simulink model "Q1Induction_Motor"  (R2013a)
settings: Solver=ode45  StartTime=0.0  StopTime=5  MaxStep=1e-4  RelTol=1e-3
settings Model: Creator=Sony  LastModifiedBy=Sony

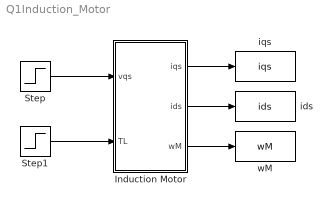
== system Q1Induction_Motor ==
  Induction Motor : Subsystem  mask{Rs=0.277, Lr=0.05606, Ls=0.0553, Lm=0.0538, La=0.0553-((0.0538*0.0538)/0.05606), J=0.0165, B=0.05, ws=2*pi*60, P=4}
      mask prompts: Rs "Rs (ohm)"; Lr "Lr (H)"; Ls "Ls (H)"; Lm "Lm (H)"; La "La (H)"; J "J (kgm^2)"; B "B (kgm^2/s)"; ws "ws (rad/s)"
  Step : Step  Time=0.1  After=200*sqrt(2)/sqrt(3)  SampleTime=0
  Step1 : Step  Time=2.5  SampleTime=0
  ids : ToWorkspace  VariableName=ids  SampleTime=-1  SaveFormat=Timeseries
  iqs : ToWorkspace  VariableName=iqs  SampleTime=-1  SaveFormat=Timeseries
  wM : ToWorkspace  VariableName=wM  SampleTime=-1  SaveFormat=Timeseries
  wires:
  Induction Motor/1(iqs) -> iqs/1
  Induction Motor/3(wM) -> wM/1
  Step/1 -> Induction Motor/1(vqs)
  Step1/1 -> Induction Motor/2(TL)
  Induction Motor/2(ids) -> ids/1

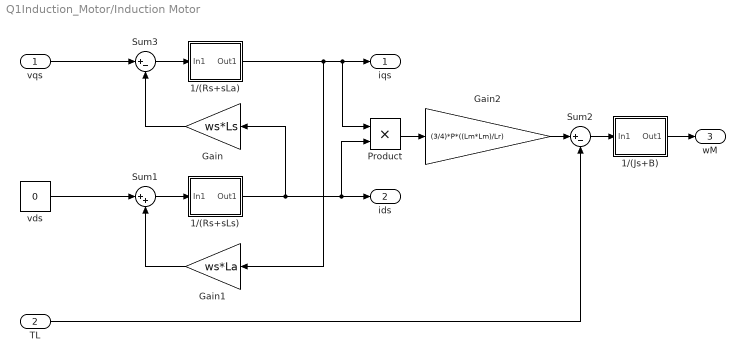
== system Q1Induction_Motor/Induction Motor ==
  vqs : Inport
  TL : Inport  Port=2
  1/(Js+B) : Subsystem  mask{J=J, B=B}
  1/(Rs+sLa) : Subsystem  mask{L=La, R=Rs}
      mask prompts: L "L (Henry)"; R "R (Ohm)"
  1/(Rs+sLs) : Subsystem  mask{L=Ls, R=Rs}
      mask prompts: L "L (Henry)"; R "R (Ohm)"
  Gain : Gain  Gain=ws*Ls
  Gain1 : Gain  Gain=ws*La
  Gain2 : Gain  Gain=(3/4)*P*((Lm*Lm)/Lr)
  Product : Product
  Sum1 : Sum  Inputs=|++
  Sum2 : Sum  Inputs=|+-
  Sum3 : Sum  Inputs=|+-
  vds : Constant  Value=0
  iqs : Outport
  ids : Outport  Port=2
  wM : Outport  Port=3
  wires:
  vqs/1 -> Sum3/1
  1/(Rs+sLs)/1(Out1) -> Gain/1, Product/2, ids/1
  Gain/1 -> Sum3/2
  vds/1 -> Sum1/1
  1/(Rs+sLa)/1(Out1) -> Gain1/1, Product/1, iqs/1
  Gain1/1 -> Sum1/2
  Sum3/1 -> 1/(Rs+sLa)/1(In1)
  Sum1/1 -> 1/(Rs+sLs)/1(In1)
  Product/1 -> Gain2/1
  Gain2/1 -> Sum2/1
  TL/1 -> Sum2/2
  Sum2/1 -> 1/(Js+B)/1(In1)
  1/(Js+B)/1(Out1) -> wM/1

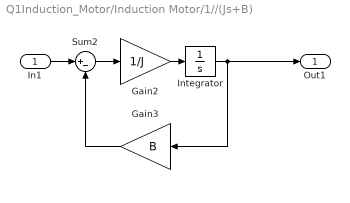
== system Q1Induction_Motor/Induction Motor/1//(Js+B) ==
  In1 : Inport
  Gain2 : Gain  Gain=1/J
  Gain3 : Gain  Gain=B
  Integrator : Integrator
  Sum2 : Sum  Inputs=|+-
  Out1 : Outport
  wires:
  Gain3/1 -> Sum2/2
  Sum2/1 -> Gain2/1
  Gain2/1 -> Integrator/1
  In1/1 -> Sum2/1
  Integrator/1 -> Out1/1, Gain3/1

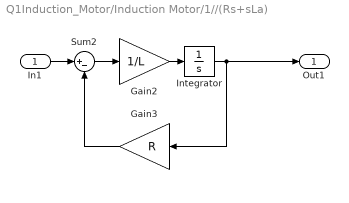
== system Q1Induction_Motor/Induction Motor/1//(Rs+sLa) ==
  In1 : Inport
  Gain2 : Gain  Gain=1/L
  Gain3 : Gain  Gain=R
  Integrator : Integrator
  Sum2 : Sum  Inputs=|+-
  Out1 : Outport
  wires:
  Gain3/1 -> Sum2/2
  Sum2/1 -> Gain2/1
  Gain2/1 -> Integrator/1
  In1/1 -> Sum2/1
  Integrator/1 -> Out1/1, Gain3/1

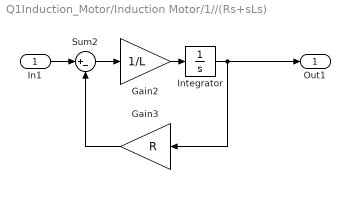
== system Q1Induction_Motor/Induction Motor/1//(Rs+sLs) ==
  In1 : Inport
  Gain2 : Gain  Gain=1/L
  Gain3 : Gain  Gain=R
  Integrator : Integrator
  Sum2 : Sum  Inputs=|+-
  Out1 : Outport
  wires:
  Gain3/1 -> Sum2/2
  Sum2/1 -> Gain2/1
  Gain2/1 -> Integrator/1
  In1/1 -> Sum2/1
  Integrator/1 -> Out1/1, Gain3/1
